simulink model "verify_ElectricConsumptionPump_mdl"  (R2018b)
settings: Solver=VariableStepDiscrete  StartTime=0.0  StopTime=20  MaxStep=0.1  RelTol=1e-3  EnableMultiTasking=on
libraries: carnot x1, simulink x1
settings Model: Creator=drhf  LastModifiedBy=drhf
settings DataIOCC: LimitDataPoints=on  SaveFormat=Array
settings OptimizationCC: ExpressionDepthLimit=2147483647  LifeSpan=inf
settings DebuggingCC: UnderspecifiedInitializationDetection=Classic  MergeDetectMultiDrivingBlocksExec=none  SolverPrmCheckMsg=warning  StateNameClashWarn=warning  SFUnexpectedBacktrackingDiag=warning  SFNoUnconditionalDefaultTransitionDiag=warning  SFExecutionAtInitializationDiag=none
settings HardwareCC: ProdBitPerPointer=32  ProdBitPerSizeT=32  ProdBitPerPtrDiffT=32  ProdLargestAtomicFloat=None  ProdIntDivRoundTo=Undefined  ProdEndianess=Unspecified  ProdWordSize=32  ProdHWDeviceType=32-bit Generic
settings ModelReferenceCC: PropagateSignalLabelsOutOfModel=off
settings SFSimCC: SimUseLocalCustomCode=off
settings RTWCC: RTWUseLocalCustomCode=off
settings CodeAppCC: StateflowObjectComments=on
settings GRTTargetCC: TargetLangStandard=C89/C90 (ANSI)  GeneratePreprocessorConditionals=Disable all  CombineOutputUpdateFcns=off  GRTInterface=on
settings ConfigComp: CovMetricSettings=dw  CovHtmlReporting=on  CovSaveCumulativeToWorkspaceVar=on  CovSaveSingleToWorkspaceVar=on  CovExternalEMLEnable=off

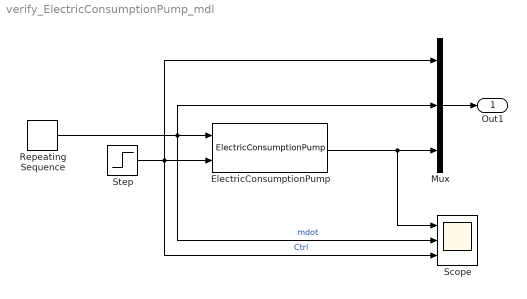
== system verify_ElectricConsumptionPump_mdl ==
  ElectricConsumptionPump : carnot/Basic/Hydraulics/ElectricConsumptionPump  e0=10  e1=20  e2=-10
  Mux : Mux  Inputs=3
  Repeating Sequence : simulink/Sources/Repeating Sequence  rep_seq_t=[0 9.9 10 20 21]  rep_seq_y=[0 1 0 1 1]
  Scope : Scope  NumInputPorts=3
  Step : Step  Time=10  SampleTime=0
  Out1 : Outport
  wires:
  Repeating Sequence/1 -> Mux/2, Scope/2, ElectricConsumptionPump/1  "mdot"
  ElectricConsumptionPump/1 -> Mux/3, Scope/1
  Step/1 -> Mux/1, Scope/3, ElectricConsumptionPump/2  "Ctrl"
  Mux/1 -> Out1/1
